simulink model "P2003_230208_FiniteTimeEstimator1"  (R2022b)
settings: Solver=VariableStepAuto  StartTime=0.0  StopTime=1  RelTol=1e-7
values from neighbouring files (symbols this model uses):
  alpha1 = Alpha1    (= 0.5)    [P2003_230210_FiniteTimeParameterEffects.m]
  alpha2 = Alpha2    (= 2.5)    [P2003_230210_FiniteTimeParameterEffects.m]
  lambda1 = Lambda1    (= 1.5)    [P2003_230210_FiniteTimeParameterEffects.m]
  lambda2 = Lambda2 + deltaLambda * (ii - 1) - deltaLambda * 2    [P2003_230210_FiniteTimeParameterEffects.m]
settings Model: PacingRate=0.130000  Creator=turib  LastModifiedBy=turib
settings HardwareCC: ProdHWDeviceType=AMD->x86-64 (Windows64)

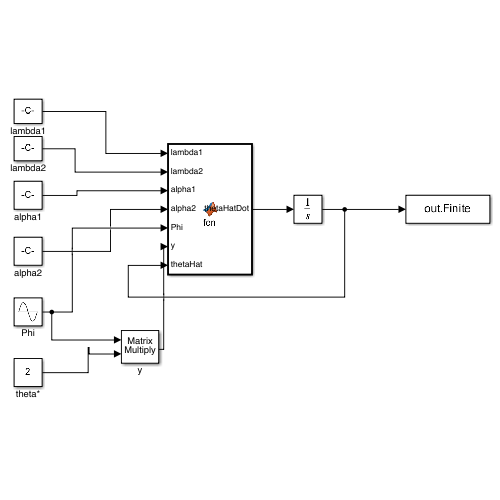
[thumbnail: Simulink's stored preview of the top-level diagram]
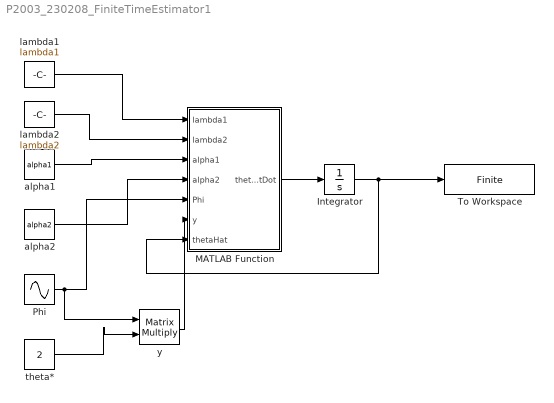
== system P2003_230208_FiniteTimeEstimator1 ==
  Integrator : Integrator
  MATLAB Function : MATLAB Function  TreatAsAtomicUnit=on
  Phi : Sin  Bias=2  SampleTime=0
  To Workspace : ToWorkspace  VariableName=Finite  SampleTime=-1
  alpha1 : Constant  Value=alpha1
  alpha2 : Constant  Value=alpha2
  lambda1 : Constant  Value=lambda1
  lambda2 : Constant  Value=lambda2
  theta* : Constant  Value=2
  y : Product  Multiplication=Matrix(*)  OutDataTypeStr=double
  wires:
  theta*/1 -> y/2
  Phi/1 -> MATLAB Function/5(Phi), y/1
  alpha1/1 -> MATLAB Function/3(alpha1)
  alpha2/1 -> MATLAB Function/4(alpha2)
  y/1 -> MATLAB Function/6(y)
  MATLAB Function/1(thetaHatDot) -> Integrator/1
  Integrator/1 -> To Workspace/1, MATLAB Function/7(thetaHat)
  lambda1/1 -> MATLAB Function/1(lambda1)
  lambda2/1 -> MATLAB Function/2(lambda2)

== matlab function P2003_230208_FiniteTimeEstimator1/MATLAB Function ==
  data: lambda1 input; thetaHatDot output; lambda2 input; alpha1 input; alpha2 input; Phi input; y input; thetaHat input
function thetaHatDot = fcn(lambda1, lambda2, alpha1, alpha2, ...
    Phi, y, thetaHat)

termNumerator = Phi' * Phi * thetaHat - Phi' * y;
termDenominator = Phi' * Phi * thetaHat - Phi' * y;
termDenominator = norm(termDenominator);
term1 = termDenominator ^ (1 - alpha1);
term1 = - lambda1 * (termNumerator / term1);
term2 = termDenominator ^ (1 - alpha2);
term2 = - lambda2 * (termNumerator / term2);
thetaHatDot = term1 + term2;

end
